simulink model "floorsignal"  (R2022a)
settings: Solver=VariableStepAuto  StartTime=0.0  StopTime=5  MaxStep=0.001  RelTol=1e-3
model workspace (MAT data in the model file):
  ltile = 0.30084
values from neighbouring files (symbols this model uses):
  Dgroove = 0.01    [SYDE351Project.m]
  Dtile = 0.3048    [SYDE351Project.m]
  Hgroove = 0.005    [SYDE351Project.m]
  speed = 1    [SYDE351Project.m]
undefined symbols (not defined in the file or in its folder): lgroove
settings Model: Creator=lanam  LastModifiedBy=lanam

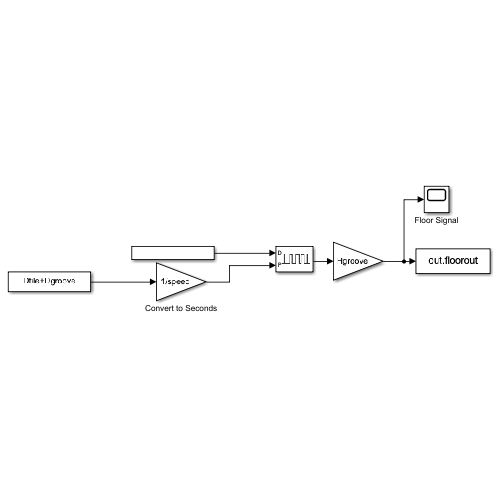
[thumbnail: Simulink's stored preview of the top-level diagram]
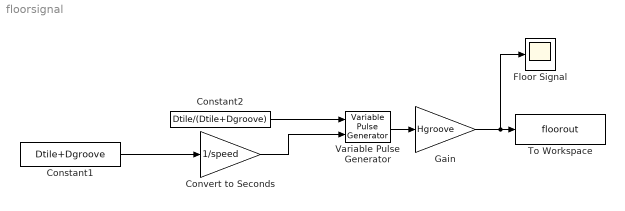
== system floorsignal ==
  Constant1 : Constant  Value=Dtile+Dgroove
  Constant2 : Constant  Value=Dtile/(Dtile+Dgroove)
  Convert to Seconds : Gain  Gain=1/speed
  Floor Signal : Scope
  Gain : Gain  Gain=Hgroove
  To Workspace : ToWorkspace  VariableName=floorout  SaveFormat=Timeseries  SampleTime=-1
  Variable Pulse Generator : VariablePulseGenerator  SampleTime=ltile + lgroove
  wires:
  Variable Pulse Generator/1 -> Gain/1
  Constant2/1 -> Variable Pulse Generator/1
  Constant1/1 -> Convert to Seconds/1
  Convert to Seconds/1 -> Variable Pulse Generator/2
  Gain/1 -> To Workspace/1, Floor Signal/1
